simulink model "main_sim_adapt_Gref_SP"  (Simulink 7.2)
settings: Solver=ode2  SolverMode=SingleTasking  StartTime=0.0  StopTime=tsim_max  FixedStep=dtsim  RelTol=1e-3
StopFcn:
  | %mkplt
values from neighbouring files (symbols this model uses):
  aero_surf_qbar_off = get_value('aero_surf_qbar_off')    [setup_claw.m]
  aero_surf_qbar_on = get_value('aero_surf_qbar_on')    [setup_claw.m]
  assertion_time = get_value('assertion_time')    [setup_sim.m]
  att_cmd_select = get_value('att_cmd_select')    [setup_sim.m]
  att_trim_IC = orientation.att'    [setup_claw.m]
  att_type_numbers = cell2mat(struct2cell(att_type))    [setup_constants.m]
  chi_trim_IC = orientation.Vchigam(2)    [setup_claw.m]
  command_time = engage_time + 2.0    [setup_sim.m]
  compute_all_rate_cols = get_value('compute_all_rate_cols')    [setup_claw.m]
  compute_all_vel_cols = get_value('compute_all_vel_cols')    [setup_claw.m]
  da_trim_IC = tmp(1)    [setup_claw.m]
  dc_L2W_IC = orientation.dc_L2W    [setup_claw.m]
  de_trim_IC = tmp(2)    [setup_claw.m]
  dr_trim_IC = tmp(3)    [setup_claw.m]
  dtsim = get_value('dtsim')    [setup_sim.m]
  E_trim_IC = MACH_pos_IC(2)    [setup_claw.m]
  Ed_trim_IC = MACH_vel_IC(2)    [setup_claw.m]
  gain_set = gain_set_next    (= 1)    [setup_claw.m]
  gain_var_struct = rmfield(gain_var_struct,setdiff(fieldnames(gain_var_struct),{'name','size'}))    [setup_claw.m]
  gamma_trim_IC = orientation.Vchigam(3)    [setup_claw.m]
  h_trim_IC = MACH_pos_IC(3)    [setup_claw.m]
  hd_trim_IC = MACH_vel_IC(3)    [setup_claw.m]
  ideal_vel_Kb = MACH_vel_Kb(1)    [setup_sim.m]
  MACH = rmfield(MACH,'vel_throt_lrlim')    [setup_claw.m]
  MACH_att_fb = get_value('MACH_att_fb','onerror',0)    [setup_claw.m]
  MACH_att_int_IC = (1-MACH_att_Kc).*MACH_quat_IC'    [setup_ideal.m]
  MACH_att_Kb = repval(att_kbnom,MACH.att_num_cv)    [setup_claw.m]
  MACH_att_Kc = Ki2Kc(MACH_att_Ki)    [setup_ideal.m]
  MACH_att_Ki = repval(att_fi,MACH.att_num_cv)    [setup_claw.m]
  MACH_gain_mat = vertcat(MACH_gain_mat, this_gain_mat)    [setup_claw.m]
  MACH_mass_IC = obac_params.mass_IC    [setup_claw.m]
  MACH_pos_IC = x_obac_IC(MACH.NEh_idx)    [setup_claw.m]
  MACH_pos_int_IC = (1-MACH_pos_Kc).*MACH_pos_IC' + MACH_vel_IC'./MACH_pos_Kb    [setup_ideal.m]
  MACH_pos_Kb = repval(pos_kbnom,MACH.pos_num_cv)    [setup_claw.m]
  MACH_pos_Kc = Ki2Kc(MACH_pos_Ki)    [setup_ideal.m]
  MACH_pos_Ki = repval(pos_fi,MACH.pos_num_cv)    [setup_claw.m]
  MACH_pqr_Bmat_IC = Bo(MACH.pqr_idx,MACH.pqr_u_idx)    [setup_claw.m]
  MACH_pqr_IC = pqr_trim_IC    [setup_claw.m]
  MACH_pqr_int_IC = (1-MACH_pqr_Kc).*MACH_pqr_IC'    [setup_ideal.m]
  MACH_pqr_Kb = repval(pqr_kbnom,MACH.pqr_num_cv)    [setup_claw.m]
  MACH_pqr_Kc = Ki2Kc(MACH_pqr_Ki)    [setup_ideal.m]
  MACH_pqr_Ki = repval(pqr_fi,MACH.pqr_num_cv)    [setup_claw.m]
  MACH_pqr_u_IC = [ vanes_trim_IC; tvc_trim_IC; rcs_trim_IC ]    [setup_claw.m]
  MACH_quat_IC = quat_trim_IC    [setup_claw.m]
  MACH_throttle_IC = throttle_trim_IC    [setup_claw.m]
  MACH_U_nom_IC = zeros(MACH.num_u,1)    [setup_claw.m]
  MACH_vel_Bmat_IC = MACH_vel_Bmat_IC*inv(vel_perts)    [setup_claw.m]
  MACH_vel_cvdnom_IC = repval(get_value('vel_cvdnom_IC','onerror',MACH_vel_cvdnom_IC),length(MACH_vel_cvdnom_IC))'    [setup_claw.m]
  MACH_vel_IC = orientation.NdEdhd'    [setup_claw.m]
  MACH_vel_int_IC = (1-MACH_vel_Kc).*MACH_vel_IC'    [setup_ideal.m]
  MACH_vel_Kb = repval(vel_kbnom,MACH.vel_num_cv)    [setup_claw.m]
  MACH_vel_Kc = Ki2Kc(MACH_vel_Ki)    [setup_ideal.m]
  MACH_vel_Ki = repval(vel_fi,MACH.vel_num_cv)    [setup_claw.m]
  MACH_vel_uold_IC = [ MACH_quat_IC; MACH_throttle_IC ]    [setup_claw.m]
  N_trim_IC = MACH_pos_IC(1)    [setup_claw.m]
  Nd_trim_IC = MACH_vel_IC(1)    [setup_claw.m]
  obac_params = define_model('obac', get_value('obac_model_type'))    [setup_claw.m]
  pos_cmd_select = get_value('pos_cmd_select')    [setup_sim.m]
  pqr_trim_IC = [ 0 0 0 ]'    [setup_claw.m]
  rate_cmd_select = get_value('rate_cmd_select')    [setup_sim.m]
  rcs_cvddes_thresh = get_value('rcs_cvddes_thresh')    [setup_claw.m]
  reset_camcmd_on_entry = get_value('reset_camcmd_on_entry')    [setup_claw.m]
  throttle_trim_IC = u_obac_IC(MACH.throttle_idx)    [setup_claw.m]
  trac_params = define_model('trac', get_value('trac_model_type','onerror',obac_params.model_type))    [setup_sim.m]
  use_auto_att_type = get_value('use_auto_att_type','onerror',0)    [setup_claw.m]
  use_eow_as_iv = get_value('use_eow_as_iv')    [setup_claw.m]
  use_full_surf_cmd = get_value('use_full_surf_cmd')    [setup_sim.m]
  use_nav = get_value('use_nav')    [setup_claw.m]
  use_NdEdh_pos = get_value('use_NdEdh_pos')    [setup_claw.m]
  use_pos_fltpath_lim = get_value('use_pos_fltpath_lim')    [setup_claw.m]
  use_throt_estimate = get_value('use_throt_estimate')    [setup_claw.m]
  use_variable_mass = get_value('use_variable_mass')    [setup_claw.m]
  use_wind_est = get_value('use_wind_est')    [setup_claw.m]
  V_trim_IC = orientation.Vchigam(1)    [setup_claw.m]
  vel_cmd_ramp_time = get_value('vel_cmd_ramp_time')    [setup_claw.m]
  vel_cmd_select = get_value('vel_cmd_select')    [setup_sim.m]
  x_trac_IC = x_obac_IC    [setup_sim.m]
undefined symbols (not defined in the file or in its folder): accel_cmd, alpha_trim, Am, att_type, B1, bb_ellipsoid, bb_params, Bm, C, constants, cosA, DiscIntNeverNeededParam, DZkx, DZtheta, E_rwy, Ed_cmd, eow_boundary, flag_autoadapt, flag_exsig, flag_uad, full_surf_llim, full_surf_ulim, gam_cmd_descent, gam_cmd_preflare, gamdot_cmd_descent, gamdot_cmd_flare, gamdot_cmd_preflare, Gamtheta, Gamx, hd_cmd, in_error_thresh, in_exsig_vecin, in_exsig_vecout, in_reset_stoptime, in_t_exsig, in_t_timer, in_tadaptoff_forced, in_tadapton_forced, Kb, Kxhat0, Kxnom, Kxstar, max_chi_cmd, max_LOS_rate, max_vel_cmd, min_chi_cmd, min_vel_cmd, modes, N_rwy, Nd_cmd, Nrbf, P, pos, Sig, sinA, target_pos_IC, target_range_blind, target_range_detect, target_range_homing, target_vel_IC ... (+11)
libraries: simulink x44, utility_lib x36, mach_lib x24, model_lib x13, simulink_need_slupdate x8, models x8
(part 6 of 8)

== system main_sim_adapt_Gref_SP/claw_main/state est/process sensors/navigation complementary filter ==
  NEh nav : Inport  OutDataType=sfix(16)  OutScaling=2^0
  NEh dot : Inport  Port=2  OutDataType=sfix(16)  OutScaling=2^0
  Gain1 : Gain  Gain=MACH.K_velpos  ParameterDataType=sfix(16)  ParameterScaling=2^0  OutDataType=sfix(16)  OutScaling=2^0  SaturateOnIntegerOverflow=on  OutDataTypeStr=Inherit: Same as input  ParamDataTypeStr=Inherit: Same as input
  Sum1 : Sum  Inputs=|+-  OutDataType=sfix(16)  OutScaling=2^0  SaturateOnIntegerOverflow=on
  Sum2 : Sum  Inputs=++|  OutDataType=sfix(16)  OutScaling=2^0  SaturateOnIntegerOverflow=on  InputSameDT=on  OutDataTypeStr=Inherit: Same as first input
  integration1 : DiscreteIntegrator  SampleTime=-1  OutDataType=sfix(16)  OutScaling=2^0  ICPrevOutput=DiscIntNeverNeededParam  ICPrevScaledInput=DiscIntNeverNeededParam
  NEh_fil : Outport  OutDataType=sfix(16)  OutScaling=2^0
  wires:
  NEh dot/1 -> Sum2/1
  NEh nav/1 -> Sum1/1
  Gain1/1 -> Sum2/2
  Sum2/1 -> integration1/1
  integration1/1 -> NEh_fil/1, Sum1/2
  Sum1/1 -> Gain1/1

== system main_sim_adapt_Gref_SP/claw_main/state est/process sensors/select e sign ==
  e in : Inport  OutDataType=sfix(16)  OutScaling=2^0
  e_past : Inport  Port=2  OutDataType=sfix(16)  OutScaling=2^0
  Dot Product : simulink/Math Operations/Dot Product  InputSameDT=on  OutDataType=sfix(16)  OutScaling=2^-10  DoSatur=off
  Gain : Gain  Gain=-1  ParameterDataType=sfix(16)  ParameterScaling=2^0  OutDataType=sfix(16)  OutScaling=2^0  SaturateOnIntegerOverflow=on  OutDataTypeStr=Inherit: Same as input  ParamDataTypeStr=Inherit: Same as input
  Switch : Switch  SaturateOnIntegerOverflow=on
  e out : Outport  OutDataType=sfix(16)  OutScaling=2^0
  wires:
  e_past/1 -> Dot Product/2
  Switch/1 -> e out/1
  Gain/1 -> Switch/3
  Dot Product/1 -> Switch/2
  e in/1 -> Gain/1, Switch/1, Dot Product/1

== system main_sim_adapt_Gref_SP/claw_main/state est/process sensors/wait for valid nav ==
  latlonh : Inport  OutDataType=sfix(16)  OutScaling=2^0
  nav_ok : Inport  Port=2  OutDataType=sfix(16)  OutScaling=2^0
  Switch3 : Switch  Threshold=0.5  SaturateOnIntegerOverflow=on
  Unit Delay1 : UnitDelay  Orientation=left  SampleTime=-1
  LLh_0 : Outport  OutDataType=sfix(16)  OutScaling=2^0
  nav_valid : Outport  Port=2  OutDataType=sfix(16)  OutScaling=2^0
  wires:
  nav_ok/1 -> nav_valid/1, Switch3/2
  latlonh/1 -> Switch3/3
  Switch3/1 -> Unit Delay1/1, LLh_0/1
  Unit Delay1/1 -> Switch3/1

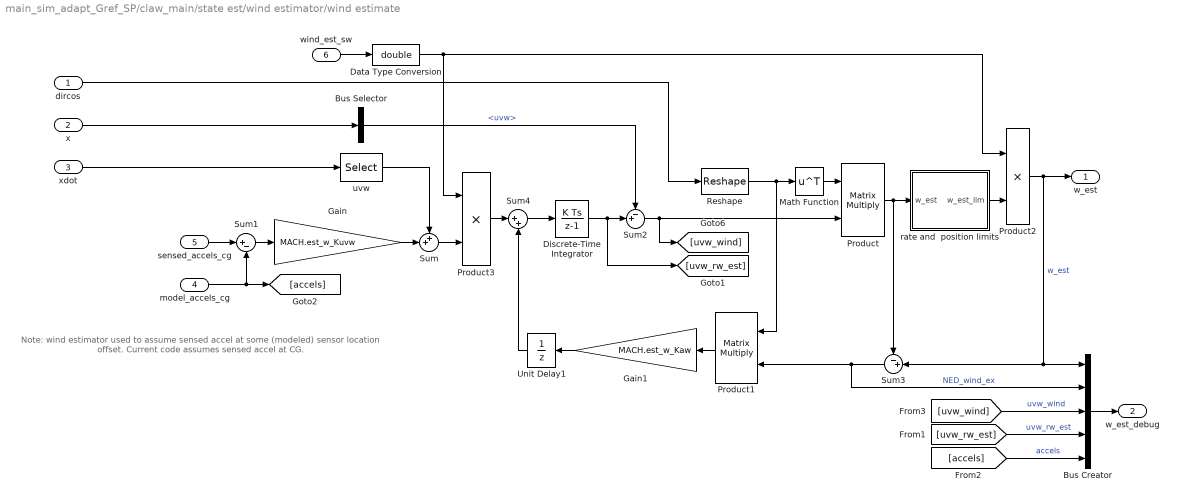
== system main_sim_adapt_Gref_SP/claw_main/state est/wind estimator/wind estimate ==
  note: Note: wind estimator used to assume sensed accel
      | at some (modeled) sensor location offset.
      |  Current code assumes sensed accel at CG.
  dircos : Inport  OutDataType=sfix(16)  OutScaling=2^0
  x : Inport  Port=2  OutDataType=sfix(16)  OutScaling=2^0
  xdot : Inport  Port=3  OutDataType=sfix(16)  OutScaling=2^0
  model_accels_cg : Inport  Port=4  OutDataType=sfix(16)  OutScaling=2^0
  sensed_accels_cg : Inport  Port=5  OutDataType=sfix(16)  OutScaling=2^0
  wind_est_sw : Inport  Port=6  OutDataType=sfix(16)  OutScaling=2^0
  Bus Creator : BusCreator  Inputs=5
  Bus Selector : BusSelector  OutputSignals=uvw
  Data Type Conversion : DataTypeConversion  OutDataTypeMode=double  OutDataType=sfix(16)  OutScaling=2^0  OutDataTypeStr=double  SaturateOnIntegerOverflow=on  RndMeth=Zero
  Discrete-Time Integrator : DiscreteIntegrator  SampleTime=-1  OutDataType=sfix(16)  OutScaling=2^0  ICPrevOutput=DiscIntNeverNeededParam  ICPrevScaledInput=DiscIntNeverNeededParam
  Gain : Gain  Gain=MACH.est_w_Kuvw  ParameterDataType=sfix(16)  ParameterScaling=2^0  OutDataType=sfix(16)  OutScaling=2^0  SaturateOnIntegerOverflow=on  OutDataTypeStr=Inherit: Same as input  ParamDataTypeStr=Inherit: Same as input
  Gain1 : Gain  Orientation=left  Gain=MACH.est_w_Kaw  ParameterDataType=sfix(16)  ParameterScaling=2^0  OutDataType=sfix(16)  OutScaling=2^0  SaturateOnIntegerOverflow=on  OutDataTypeStr=Inherit: Same as input  ParamDataTypeStr=Inherit: Same as input
  Math Function : Math  Operator=transpose  OutDataType=sfix(16)  OutScaling=2^0  SaturateOnIntegerOverflow=on
  Product : Product  Multiplication=Matrix(*)  OutDataType=sfix(16)  OutScaling=2^0  SaturateOnIntegerOverflow=on  OutDataTypeStr=Inherit: Same as first input
  Product1 : Product  Orientation=left  Multiplication=Matrix(*)  OutDataType=sfix(16)  OutScaling=2^0  SaturateOnIntegerOverflow=on  OutDataTypeStr=Inherit: Same as first input
  Product2 : Product  OutDataType=sfix(16)  OutScaling=2^0  SaturateOnIntegerOverflow=on  OutDataTypeStr=Inherit: Same as first input
  Product3 : Product  OutDataType=sfix(16)  OutScaling=2^0  SaturateOnIntegerOverflow=on  OutDataTypeStr=Inherit: Same as first input
  Reshape : Reshape  OutputDimensionality=Customize  OutputDimensions=[3,3]
  Sum : Sum  Inputs=++|  OutDataType=sfix(16)  OutScaling=2^0  SaturateOnIntegerOverflow=on  InputSameDT=on  OutDataTypeStr=Inherit: Same as first input
  Sum1 : Sum  Inputs=|+-  OutDataType=sfix(16)  OutScaling=2^0  SaturateOnIntegerOverflow=on  InputSameDT=on  OutDataTypeStr=Inherit: Same as first input
  Sum2 : Sum  Inputs=-+|  OutDataType=sfix(16)  OutScaling=2^0  SaturateOnIntegerOverflow=on
  Sum3 : Sum  Orientation=left  Inputs=-+|  OutDataType=sfix(16)  OutScaling=2^0  SaturateOnIntegerOverflow=on
  Sum4 : Sum  Inputs=|++  OutDataType=sfix(16)  OutScaling=2^0  SaturateOnIntegerOverflow=on  InputSameDT=on  OutDataTypeStr=Inherit: Same as first input
  Unit Delay1 : UnitDelay  Orientation=left  X0=zeros(3,1)  SampleTime=-1
  rate and  position limits : Subsystem
  uvw : Selector  InputPortWidth=MACH.num_x  IndexOptions=Index vector (dialog)  Indices=MACH.uvw_idx  OutputSizes=1
  w_est : Outport  OutDataType=sfix(16)  OutScaling=2^0
  w_est_debug : Outport  Port=2  OutDataType=sfix(16)  OutScaling=2^0
  wires:
  Discrete-Time Integrator/1 -> Sum2/2, [uvw_rw_est]
  sensed_accels_cg/1 -> Sum1/1
  Sum1/1 -> Gain/1
  Sum/1 -> Product3/2
  Gain/1 -> Sum/2
  Bus Selector/1 -> Sum2/1  "<uvw>"
  dircos/1 -> Reshape/1
  Reshape/1 -> Math Function/1, Product1/1
  Product/1 -> Sum3/1, rate and  position limits/1(w_est)
  Math Function/1 -> Product/1
  Sum2/1 -> Product/2, [uvw_wind]
  Gain1/1 -> Unit Delay1/1
  xdot/1 -> uvw/1
  uvw/1 -> Sum/1
  x/1 -> Bus Selector/1
  rate and  position limits/1(w_est_lim) -> Product2/2
  Product1/1 -> Gain1/1
  Sum3/1 -> Product1/2, Bus Creator/2  "NED_wind_ex"
  Product2/1 -> w_est/1, Sum3/2, Bus Creator/1  "w_est"
  wind_est_sw/1 -> Data Type Conversion/1
  Sum4/1 -> Discrete-Time Integrator/1
  Product3/1 -> Sum4/1
  Unit Delay1/1 -> Sum4/2
  Data Type Conversion/1 -> Product2/1, Product3/1
  [uvw_wind] -> Bus Creator/3  "uvw_wind"
  [uvw_rw_est] -> Bus Creator/4  "uvw_rw_est"
  [accels] -> Bus Creator/5  "accels"
  Bus Creator/1 -> w_est_debug/1
  model_accels_cg/1 -> Sum1/2, [accels]

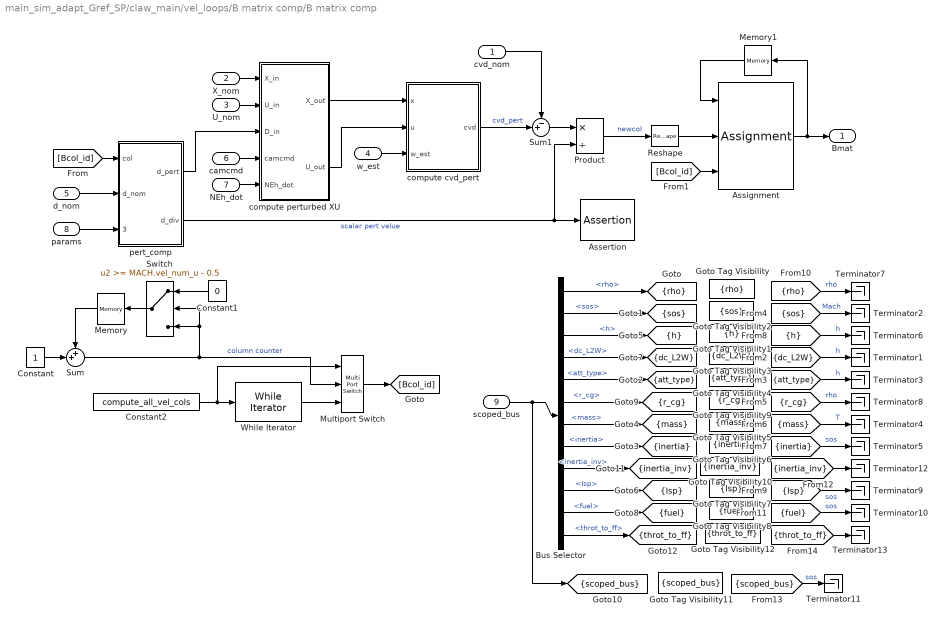
== system main_sim_adapt_Gref_SP/claw_main/vel_loops/B matrix comp/B matrix comp ==
  cvd_nom : Inport  OutDataType=sfix(16)  OutScaling=2^0
  X_nom : Inport  Port=2  OutDataType=sfix(16)  OutScaling=2^0
  U_nom : Inport  Port=3  OutDataType=sfix(16)  OutScaling=2^0
  w_est : Inport  Port=4  OutDataType=sfix(16)  OutScaling=2^0
  d_nom : Inport  Port=5  OutDataType=sfix(16)  OutScaling=2^0
  camcmd : Inport  Port=6  OutDataType=sfix(16)  OutScaling=2^0
  NEh_dot : Inport  Port=7  OutDataType=sfix(16)  OutScaling=2^0
  params : Inport  Port=8  OutDataType=sfix(16)  OutScaling=2^0
  scoped_bus : Inport  Port=9  OutDataType=sfix(16)  OutScaling=2^0
  Assertion : Assertion  Enabled=on
  Assignment : Assignment  NumberOfDimensions=2  IndexOptions=Assign all,Index vector (port)  Indices=-1,1  OutputSizes=1,1
  Bus Selector : BusSelector  OutputSignals=atmos_env.rho,atmos_env.sos,atmos_env.h,dc_L2W,att_type,mass_props.r_cg,mass_props.mass,mass_props.inertia,mass_props.inertia_inv,mass_props.Isp,mass_props.fuel,mass_props.throt_to_ff
  Constant : Constant  OutDataType=sfix(16)  OutScaling=2^0
  Constant1 : Constant  Orientation=left  Value=0  OutDataType=sfix(16)  OutScaling=2^0
  Constant2 : Constant  Value=compute_all_vel_cols  OutDataType=sfix(16)  OutScaling=2^0
  Goto Tag Visibility : GotoTagVisibility  GotoTag=rho
  Goto Tag Visibility1 : GotoTagVisibility  GotoTag=h
  Goto Tag Visibility10 : GotoTagVisibility  GotoTag=inertia_inv
  Goto Tag Visibility11 : GotoTagVisibility  GotoTag=scoped_bus
  Goto Tag Visibility12 : GotoTagVisibility  GotoTag=throt_to_ff
  Goto Tag Visibility2 : GotoTagVisibility  GotoTag=sos
  Goto Tag Visibility3 : GotoTagVisibility  GotoTag=dc_L2W
  Goto Tag Visibility4 : GotoTagVisibility  GotoTag=att_type
  Goto Tag Visibility5 : GotoTagVisibility  GotoTag=mass
  Goto Tag Visibility6 : GotoTagVisibility  GotoTag=inertia
  Goto Tag Visibility7 : GotoTagVisibility  GotoTag=Isp
  Goto Tag Visibility8 : GotoTagVisibility  GotoTag=fuel
  Goto Tag Visibility9 : GotoTagVisibility  GotoTag=r_cg
  Memory : Memory  Orientation=left  InheritSampleTime=on
  Memory1 : Memory  Orientation=left  X0=MACH_vel_Bmat_IC  InheritSampleTime=on
  Multiport Switch : MultiPortSwitch  Inputs=2  zeroidx=on
  Product : Product  Inputs=*/  OutDataType=sfix(16)  OutScaling=2^0  SaturateOnIntegerOverflow=on  InputSameDT=on  OutDataTypeStr=Inherit: Same as first input
  Reshape : Reshape  OutputDimensionality=Column vector (2-D)
  Sum : Sum  Inputs=++|  OutDataType=sfix(16)  OutScaling=2^0  SaturateOnIntegerOverflow=on  InputSameDT=on  OutDataTypeStr=Inherit: Same as first input
  Sum1 : Sum  Inputs=-+|  OutDataType=sfix(16)  OutScaling=2^0  SaturateOnIntegerOverflow=on  InputSameDT=on  OutDataTypeStr=Inherit: Same as first input
  Switch : Switch  Orientation=left  Threshold=MACH.vel_num_u - 0.5  SaturateOnIntegerOverflow=on  InputSameDT=on
  Terminator{1..13} (13 alike) : Terminator
  While Iterator : WhileIterator  MaxIters=MACH.vel_num_u  WhileBlockType=do-while  ShowIterationPort=on
  compute cvd_pert : Subsystem
  compute perturbed XU : Subsystem
  pert_comp : Subsystem
  Bmat : Outport  OutDataType=sfix(16)  OutScaling=2^0
  tag scope: Isp=scoped, att_type=scoped, dc_L2W=scoped, fuel=scoped, h=scoped, inertia=scoped, inertia_inv=scoped, mass=scoped, r_cg=scoped, rho=scoped, scoped_bus=scoped, sos=scoped, throt_to_ff=scoped
  wires:
  U_nom/1 -> compute perturbed XU/2(U_in)
  X_nom/1 -> compute perturbed XU/1(X_in)
  Product/1 -> Reshape/1  "newcol"
  Sum1/1 -> Product/1
  [Bcol_id] -> Assignment/3
  Reshape/1 -> Assignment/2
  Assignment/1 -> Bmat/1, Memory1/1
  [Bcol_id] -> pert_comp/1(col)
  d_nom/1 -> pert_comp/2(d_nom)
  pert_comp/2(d_div) -> Product/2, Assertion/1  "scalar pert value"
  pert_comp/1(d_pert) -> compute perturbed XU/3(D_in)
  w_est/1 -> compute cvd_pert/3(w_est)
  camcmd/1 -> compute perturbed XU/4(camcmd)
  NEh_dot/1 -> compute perturbed XU/5(NEh_dot)
  compute perturbed XU/1(X_out) -> compute cvd_pert/1(x)
  params/1 -> pert_comp/3(params)
  compute perturbed XU/2(U_out) -> compute cvd_pert/2(u)
  Memory1/1 -> Assignment/1
  scoped_bus/1 -> Bus Selector/1, [scoped_bus]
  [rho] -> Terminator7/1  "rho"
  [sos] -> Terminator2/1  "Mach"
  [h] -> Terminator6/1  "h"
  Bus Selector/1 -> [rho]  "<rho>"
  Bus Selector/2 -> [sos]  "<sos>"
  Bus Selector/3 -> [h]  "<h>"
  [dc_L2W] -> Terminator1/1  "h"
  Bus Selector/4 -> [dc_L2W]  "<dc_L2W>"
  Constant2/1 -> Multiport Switch/1, While Iterator/1
  While Iterator/1 -> Multiport Switch/3
  Constant1/1 -> Switch/1
  Sum/1 -> Switch/3, Switch/2, Multiport Switch/2  "column counter"
  Switch/1 -> Memory/1
  Memory/1 -> Sum/1
  Constant/1 -> Sum/2
  Multiport Switch/1 -> [Bcol_id]
  [att_type] -> Terminator3/1  "h"
  Bus Selector/5 -> [att_type]  "<att_type>"
  [r_cg] -> Terminator8/1  "rho"
  [mass] -> Terminator4/1  "T"
  [inertia] -> Terminator5/1  "sos"
  Bus Selector/6 -> [r_cg]  "<r_cg>"
  Bus Selector/7 -> [mass]  "<mass>"
  Bus Selector/8 -> [inertia]  "<inertia>"
  [Isp] -> Terminator9/1  "sos"
  Bus Selector/10 -> [Isp]  "<Isp>"
  [fuel] -> Terminator10/1  "sos"
  Bus Selector/11 -> [fuel]  "<fuel>"
  compute cvd_pert/1(cvd) -> Sum1/2  "cvd_pert"
  cvd_nom/1 -> Sum1/1
  [inertia_inv] -> Terminator12/1
  Bus Selector/9 -> [inertia_inv]  "<inertia_inv>"
  [scoped_bus] -> Terminator11/1  "sos"
  Bus Selector/12 -> [throt_to_ff]  "<throt_to_ff>"
  [throt_to_ff] -> Terminator13/1

== system main_sim_adapt_Gref_SP/claw_main/vel_loops/B matrix comp/compute cvd_nom ==
  note: Note: this computation of NEh accelerations
      | assumes that pqr = 0
  x : Inport  OutDataType=sfix(16)  OutScaling=2^0
  u : Inport  Port=2  OutDataType=sfix(16)  OutScaling=2^0
  w_est : Inport  Port=3  OutDataType=sfix(16)  OutScaling=2^0
  Bus Selector : BusSelector  OutputSignals=dircos
  Gain : Gain  Gain=[1 1 -1]  ParameterDataType=sfix(16)  ParameterScaling=2^0  OutDataType=sfix(16)  OutScaling=2^0  SaturateOnIntegerOverflow=on  OutDataTypeStr=Inherit: Same as input  ParamDataTypeStr=Inherit: Same as input
  Math Function : Math  Operator=transpose  OutDataType=sfix(16)  OutScaling=2^0  SaturateOnIntegerOverflow=on
  Product : Product  Multiplication=Matrix(*)  OutDataType=sfix(16)  OutScaling=2^0  SaturateOnIntegerOverflow=on  InputSameDT=on  OutDataTypeStr=Inherit: Same as first input
  Reshape : Reshape  OutputDimensionality=Customize  OutputDimensions=[3,3]
  cl model : models/gtm-obac  SystemSampleTime=-1
  uvw_dot : Selector  InputPortWidth=MACH.num_x  IndexOptions=Index vector (dialog)  Indices=MACH.uvw_idx  OutputSizes=1
  cvd : Outport  OutDataType=sfix(16)  OutScaling=2^0
  wires:
  uvw_dot/1 -> Product/2
  x/1 -> cl model/1
  Reshape/1 -> Math Function/1
  Math Function/1 -> Product/1
  Product/1 -> Gain/1
  Gain/1 -> cvd/1
  Bus Selector/1 -> Reshape/1  "<dircos>"
  u/1 -> cl model/2
  w_est/1 -> cl model/3
  cl model/1 -> uvw_dot/1
  cl model/2 -> Bus Selector/1

== system main_sim_adapt_Gref_SP/claw_main/vel_loops/B matrix comp/compute nominal XU ==
  X_in : Inport  OutDataType=sfix(16)  OutScaling=2^0
  U_in : Inport  Port=2  OutDataType=sfix(16)  OutScaling=2^0
  D_in : Inport  Port=3  OutDataType=sfix(16)  OutScaling=2^0
  camcmd : Inport  Port=4  OutDataType=sfix(16)  OutScaling=2^0
  NEh_dot : Inport  Port=5  OutDataType=sfix(16)  OutScaling=2^0
  Assignment1 : Assignment  IndexOptions=Index vector (dialog)  Indices=MACH.throttle_idx  OutputSizes=[1 1]
  Assignment2 : Assignment  IndexOptions=Index vector (dialog)  Indices=[ MACH.quat_idx MACH.uvw_idx]  OutputSizes=[1 1]
  Demux1 : Demux  Outputs=[ 2 MACH.num_u_throt ]
  Gain : Gain  Gain=[1 1 -1]  ParameterDataType=sfix(16)  ParameterScaling=2^0  OutDataType=sfix(16)  OutScaling=2^0  SaturateOnIntegerOverflow=on  OutDataTypeStr=Inherit: Same as input  ParamDataTypeStr=Inherit: Same as input
  Mux : Mux  Inputs=[ 2 1 ]
  Mux1 : Mux  Inputs=2
  Product1 : Product  Multiplication=Matrix(*)  OutDataType=sfix(16)  OutScaling=2^0  SaturateOnIntegerOverflow=on  OutDataTypeStr=Inherit: Same as first input
  Reshape1 : Reshape  OutputDimensionality=Customize  OutputDimensions=[3,3]
  Selector1 : Selector  InputPortWidth=MACH.num_x  IndexOptions=Index vector (dialog)  Indices=MACH.quat_idx  OutputSizes=1
  att2dc : utility_lib/att2dc  SystemSampleTime=-1
  dc2e_ref : utility_lib/dc2e_ref  SystemSampleTime=-1
  X_out : Outport  OutDataType=sfix(16)  OutScaling=2^0
  U_out : Outport  Port=2  OutDataType=sfix(16)  OutScaling=2^0
  wires:
  Mux/1 -> att2dc/1
  Demux1/2 -> Assignment1/2  "throttle"
  D_in/1 -> Demux1/1
  U_in/1 -> Assignment1/1
  X_in/1 -> Assignment2/1, Selector1/1
  Assignment1/1 -> U_out/1
  camcmd/1 -> Mux/2
  Demux1/1 -> Mux/1
  NEh_dot/1 -> Gain/1
  Reshape1/1 -> Product1/1
  Assignment2/1 -> X_out/1
  att2dc/1 -> Reshape1/1, dc2e_ref/1
  dc2e_ref/1 -> Mux1/1  "e"
  Gain/1 -> Product1/2  "NED_dot"
  Selector1/1 -> dc2e_ref/2
  Product1/1 -> Mux1/2  "uvw"
  Mux1/1 -> Assignment2/2

== system main_sim_adapt_Gref_SP/claw_main/vel_loops/convert accel_cmd to NED_dd_cmd/NED_dd cmd ==
  NEH_dd_cmd_in : Inport  OutDataType=sfix(16)  OutScaling=2^0
  Action Port : ActionPort  ActionType=case
  NEh_dd_cmd : Outport  OutDataType=sfix(16)  OutScaling=2^0  InitialOutput=zeros(3,1)
  wires:
  NEH_dd_cmd_in/1 -> NEh_dd_cmd/1

== system main_sim_adapt_Gref_SP/claw_main/vel_loops/convert accel_cmd to NED_dd_cmd/vchigam_dot cmd ==
  vchigam_dot_cmd : Inport  OutDataType=sfix(16)  OutScaling=2^0
  NEh_d : Inport  Port=2  OutDataType=sfix(16)  OutScaling=2^0
  Action Port : ActionPort  ActionType=case
  Math Function : Math  Operator=transpose  OutDataType=sfix(16)  OutScaling=2^0  SaturateOnIntegerOverflow=on
  Product2 : Product  Multiplication=Matrix(*)  OutDataType=sfix(16)  OutScaling=2^0  RndMeth=Zero
  Reshape1 : Reshape  OutputDimensionality=Customize  OutputDimensions=[3 3]
  convert to NED_d : Gain  Gain=[1 1 -1]  ParameterDataType=sfix(16)  ParameterScaling=2^0  OutDataType=sfix(16)  OutScaling=2^0
  convert to NEh_dd : Gain  Gain=[1 1 -1]  ParameterDataType=sfix(16)  ParameterScaling=2^0  OutDataType=sfix(16)  OutScaling=2^0
  polar to cart : Subsystem
  vec2dc : utility_lib/vec2dc  SystemSampleTime=-1
  NEh_dd_cmd : Outport  OutDataType=sfix(16)  OutScaling=2^0  InitialOutput=zeros(3,1)
  wires:
  vec2dc/1 -> Reshape1/1
  Reshape1/1 -> Math Function/1
  convert to NED_d/1 -> vec2dc/1
  polar to cart/1(along_dd;cross_dd;vert_dd) -> Product2/2
  NEh_d/1 -> convert to NED_d/1
  Product2/1 -> convert to NEh_dd/1
  convert to NEh_dd/1 -> NEh_dd_cmd/1
  Math Function/1 -> Product2/1
  vchigam_dot_cmd/1 -> polar to cart/2(vchigam_dot_cmd)
  vec2dc/2 -> polar to cart/1(scaling_info)

== system main_sim_adapt_Gref_SP/claw_main/vel_loops/set di params/att limits ==
  uvw : Inport  OutDataType=sfix(16)  OutScaling=2^0
  Bus Creator : BusCreator
  Constant : Constant  Value=MACH.vel_att_ulim  VectorParams1D=off  OutDataType=sfix(16)  OutScaling=2^0
  Constant1 : Constant  Value=MACH.vel_att_lrlim  OutDataType=sfix(16)  OutScaling=2^0
  Constant2 : Constant  Value=MACH.vel_att_urlim  OutDataType=sfix(16)  OutScaling=2^0
  Constant3 : Constant  Value=MACH.az_ulim  OutDataType=sfix(16)  OutScaling=2^0
  Constant7 : Constant  Value=MACH.vel_att_llim  VectorParams1D=off  OutDataType=sfix(16)  OutScaling=2^0
  Constant8 : Constant  Value=MACH.az_llim  OutDataType=sfix(16)  OutScaling=2^0
  Reshape1 : Reshape
  Reshape3 : Reshape
  Selector1 : Selector  NumberOfDimensions=2  InputPortWidth=3  IndexOptions=Index vector (port),Select all  Indices=1,-1  OutputSizes=1
  Selector2 : Selector  NumberOfDimensions=2  InputPortWidth=3  IndexOptions=Index vector (port),Select all  Indices=1,-1  OutputSizes=1
  velocity based angular rate llim : mach_lib/velocity based angular rate limit  SystemSampleTime=-1  q_idx=2
  velocity based angular rate ulim : mach_lib/velocity based angular rate limit  SystemSampleTime=-1  q_idx=2
  att_limits : Outport  OutDataType=sfix(16)  OutScaling=2^0
  wires:
  [att_type] -> Selector1/2, Selector2/2
  Constant/1 -> Selector1/1
  Constant7/1 -> Selector2/1
  Selector1/1 -> Reshape1/1
  Selector2/1 -> Reshape3/1
  Reshape1/1 -> Bus Creator/1  "att_ulim"
  Reshape3/1 -> Bus Creator/2  "att_llim"
  Constant2/1 -> velocity based angular rate ulim/1
  Constant8/1 -> velocity based angular rate ulim/2
  Constant1/1 -> velocity based angular rate llim/1
  Constant3/1 -> velocity based angular rate llim/2
  uvw/1 -> velocity based angular rate ulim/3, velocity based angular rate llim/3
  velocity based angular rate ulim/1 -> Bus Creator/3  "att_urlim"
  velocity based angular rate llim/1 -> Bus Creator/4  "att_lrlim"
  Bus Creator/1 -> att_limits/1

== system main_sim_adapt_Gref_SP/claw_main/vel_loops/set di params/combine limits ==
  att_limits : Inport  OutDataType=sfix(16)  OutScaling=2^0
  throt_limits : Inport  Port=2  OutDataType=sfix(16)  OutScaling=2^0
  Bus Creator : BusCreator
  Bus Selector : BusSelector  OutputSignals=att_ulim,att_llim,att_urlim,att_lrlim
  Bus Selector1 : BusSelector  OutputSignals=throt_ulim,throt_llim,throt_urlim,throt_lrlim
  Mux{,1..3} (4 alike) : Mux  Inputs=2
  vel_u_limits : Outport  OutDataType=sfix(16)  OutScaling=2^0
  wires:
  att_limits/1 -> Bus Selector/1
  throt_limits/1 -> Bus Selector1/1
  Bus Selector/1 -> Mux/1  "<att_ulim>"
  Bus Selector/2 -> Mux1/1  "<att_llim>"
  Bus Selector/3 -> Mux2/1  "<att_urlim>"
  Bus Selector/4 -> Mux3/1  "<att_lrlim>"
  Bus Selector1/1 -> Mux/2  "<throt_ulim>"
  Bus Selector1/2 -> Mux1/2  "<throt_llim>"
  Bus Selector1/3 -> Mux2/2  "<throt_urlim>"
  Bus Selector1/4 -> Mux3/2  "<throt_lrlim>"
  Mux/1 -> Bus Creator/1  "u_ulim"
  Mux1/1 -> Bus Creator/2  "u_llim"
  Mux2/1 -> Bus Creator/3  "u_urlim"
  Mux3/1 -> Bus Creator/4  "u_lrlim"
  Bus Creator/1 -> vel_u_limits/1

== system main_sim_adapt_Gref_SP/claw_main/vel_loops/set di params/compute dc_fltpath ==
  NEh_dot_fltpath : Inport  OutDataType=sfix(16)  OutScaling=2^0
  Gain : Gain  Gain=repmat([1 1 -1],3,1)  ParameterDataType=sfix(16)  ParameterScaling=2^0  OutDataType=sfix(16)  OutScaling=2^0
  Gain1 : Gain  Gain=[1 1 -1]  ParameterDataType=sfix(16)  ParameterScaling=2^0  OutDataType=sfix(16)  OutScaling=2^0
  Reshape : Reshape  OutputDimensionality=Customize  OutputDimensions=[3 3]
  Terminator : Terminator
  vec2dc : utility_lib/vec2dc  SystemSampleTime=-1
  dc_fltpath : Outport  OutDataType=sfix(16)  OutScaling=2^0
  wires:
  vec2dc/1 -> Reshape/1
  Reshape/1 -> Gain/1
  Gain1/1 -> vec2dc/1
  vec2dc/2 -> Terminator/1
  Gain/1 -> dc_fltpath/1
  NEh_dot_fltpath/1 -> Gain1/1

== system main_sim_adapt_Gref_SP/claw_main/vel_loops/set di params/throttle limits ==
  full_surf : Inport  OutDataType=sfix(16)  OutScaling=2^0
  throt_old : Inport  Port=2  OutDataType=sfix(16)  OutScaling=2^0
  Bus Creator : BusCreator
  Bus Selector1 : BusSelector  OutputSignals=full_surf_ulim,full_surf_llim,full_surf_urlim,full_surf_lrlim
  Selector{1..2,5..6} (4 alike) : Selector  InputPortWidth=MACH.num_u  IndexOptions=Index vector (dialog)  Indices=MACH.throttle_idx  OutputSizes=1
  rate limit limits : mach_lib/rate limit limits  SystemSampleTime=-1  ulim=MACH.vel_throt_ulim  llim=MACH.vel_throt_llim
  throt_limits : Outport  OutDataType=sfix(16)  OutScaling=2^0
  wires:
  Bus Selector1/1 -> Selector5/1  "<full_surf_ulim>"
  Bus Selector1/2 -> Selector6/1  "<full_surf_llim>"
  full_surf/1 -> Bus Selector1/1
  throt_old/1 -> rate limit limits/1
  Selector5/1 -> rate limit limits/2
  Selector6/1 -> rate limit limits/3
  Bus Creator/1 -> throt_limits/1
  rate limit limits/1 -> Bus Creator/1  "throt_ulim"
  rate limit limits/2 -> Bus Creator/2  "throt_llim"
  Bus Selector1/3 -> Selector1/1  "<full_surf_urlim>"
  Bus Selector1/4 -> Selector2/1  "<full_surf_lrlim>"
  Selector1/1 -> rate limit limits/4, Bus Creator/3  "throt_urlim"
  Selector2/1 -> rate limit limits/5, Bus Creator/4  "throt_lrlim"

== system main_sim_adapt_Gref_SP/control input (modified)/control input/form control input/add effector control params ==
  full_surf_cmd : Inport  OutDataType=sfix(16)  OutScaling=2^0
  Bus Creator : BusCreator  Inputs=9
  From Workspace : FromWorkspace  VariableName=full_surf_limits_fw.obac.ulim  SampleTime=MACH.dt  Interpolate=off  OutputAfterFinalValue=Holding final value
  From Workspace1 : FromWorkspace  VariableName=full_surf_limits_fw.obac.llim  SampleTime=MACH.dt  Interpolate=off  OutputAfterFinalValue=Holding final value
  From Workspace2 : FromWorkspace  VariableName=full_surf_limits_fw.obac.limit_select  SampleTime=MACH.dt  Interpolate=off  OutputAfterFinalValue=Holding final value
  From Workspace3 : FromWorkspace  VariableName=full_surf_limits_fw.obac.urlim  SampleTime=MACH.dt  Interpolate=off  OutputAfterFinalValue=Holding final value
  From Workspace4 : FromWorkspace  VariableName=full_surf_limits_fw.obac.lrlim  SampleTime=MACH.dt  Interpolate=off  OutputAfterFinalValue=Holding final value
  From Workspace5 : FromWorkspace  VariableName=full_surf_limits_fw.obac.pref_select  SampleTime=MACH.dt  Interpolate=off  OutputAfterFinalValue=Holding final value
  From Workspace6 : FromWorkspace  VariableName=full_surf_limits_fw.obac.pref  SampleTime=MACH.dt  Interpolate=off  OutputAfterFinalValue=Holding final value
  From Workspace7 : FromWorkspace  VariableName=full_surf_limits_fw.obac.pref_wght  SampleTime=MACH.dt  Interpolate=off  OutputAfterFinalValue=Holding final value
  full_surf : Outport  OutDataType=sfix(16)  OutScaling=2^0
  wires:
  From Workspace1/1 -> Bus Creator/3  "full_surf_llim"
  From Workspace/1 -> Bus Creator/2  "full_surf_ulim"
  full_surf_cmd/1 -> Bus Creator/1  "full_surf_cmd"
  Bus Creator/1 -> full_surf/1
  From Workspace3/1 -> Bus Creator/4  "full_surf_urlim"
  From Workspace4/1 -> Bus Creator/5  "full_surf_lrlim"
  From Workspace2/1 -> Bus Creator/6  "full_surf_lock"
  From Workspace5/1 -> Bus Creator/7  "full_surf_pref_select"
  From Workspace6/1 -> Bus Creator/8  "full_surf_pref"
  From Workspace7/1 -> Bus Creator/9  "full_surf_pref_wght"

== system main_sim_adapt_Gref_SP/control input (modified)/control input/form control input/engine parameters ==
  Bus Creator2 : BusCreator  Inputs=3
  Constant : Constant  Value=obac_params.Isp_sl  OutDataType=sfix(16)  OutScaling=2^0
  Constant1 : Constant  Value=obac_params.Isp_vacuum  OutDataType=sfix(16)  OutScaling=2^0
  Constant2 : Constant  Value=obac_params.throt_to_ff  OutDataType=sfix(16)  OutScaling=2^0
  engines : Outport  OutDataType=sfix(16)  OutScaling=2^0
  wires:
  Constant1/1 -> Bus Creator2/2  "Isp_vacuum"
  Constant/1 -> Bus Creator2/1  "Isp_sl"
  Bus Creator2/1 -> engines/1
  Constant2/1 -> Bus Creator2/3  "throt_to_ff"

== system main_sim_adapt_Gref_SP/control input (modified)/control input/form control input/mode switches ==
  control_input : Inport  OutDataType=sfix(16)  OutScaling=2^0
  Bus Creator1 : BusCreator  Inputs=17
  Bus Selector4 : BusSelector  OutputSignals=CLAW_mode,accel_submode
  Compare To Zero : simulink/Logic and Bit Operations/Compare To Zero  SystemSampleTime=-1  relop=>  LogicOutDataTypeMode=boolean  ZeroCross=off
  Data Type Conversion : DataTypeConversion  OutDataType=sfix(16)  OutScaling=2^0
  From Workspace : FromWorkspace  VariableName=enable_bb_fw  SampleTime=MACH.dt  Interpolate=off  OutputAfterFinalValue=Holding final value
  From Workspace1 : FromWorkspace  VariableName=use_att_rate_cmd_fw  SampleTime=MACH.dt  Interpolate=off  OutputAfterFinalValue=Holding final value
  From Workspace2 : FromWorkspace  VariableName=use_cam_rate_cmd_fw  SampleTime=MACH.dt  Interpolate=off  OutputAfterFinalValue=Holding final value
  From Workspace3 : FromWorkspace  VariableName=enable_homing_fw  SampleTime=MACH.dt  Interpolate=off  OutputAfterFinalValue=Holding final value
  From Workspace4 : FromWorkspace  VariableName=nav_enable_fw  SampleTime=MACH.dt  Interpolate=off  OutputAfterFinalValue=Holding final value
  From Workspace5 : FromWorkspace  VariableName=gain_set_fw  SampleTime=MACH.dt  Interpolate=off  OutputAfterFinalValue=Holding final value
  From Workspace6 : FromWorkspace  VariableName=att_type_fw  SampleTime=MACH.dt  Interpolate=off  OutputAfterFinalValue=Holding final value
  From Workspace7 : FromWorkspace  VariableName=use_held_aero_obac_fw  SampleTime=MACH.dt  Interpolate=off  OutputAfterFinalValue=Holding final value
  int_reset_sw : Constant  Value=0  OutDataType=sfix(16)  OutScaling=2^0
  llh_input_sw : Constant  Value=0  OutDataType=sfix(16)  OutScaling=2^0
  pre_takeoff_sw : Constant  Value=0  OutDataType=sfix(16)  OutScaling=2^0
  reset_pos_sw : Constant  Value=0  OutDataType=sfix(16)  OutScaling=2^0
  use_full_surf_cmd_sw : Constant  Value=use_full_surf_cmd  OutDataType=sfix(16)  OutScaling=2^0
  wind_est_sw : Constant  Value=0  OutDataType=sfix(16)  OutScaling=2^0
  mode_sw : Outport  OutDataType=sfix(16)  OutScaling=2^0
  wires:
  reset_pos_sw/1 -> Bus Creator1/5  "reset_pos_sw"
  wind_est_sw/1 -> Bus Creator1/6  "wind_est_sw"
  llh_input_sw/1 -> Bus Creator1/7  "llh_input_sw"
  Compare To Zero/1 -> Data Type Conversion/1  "engaged_sw"
  pre_takeoff_sw/1 -> Bus Creator1/4  "pre_takeoff_sw"
  int_reset_sw/1 -> Bus Creator1/8  "int_reset_sw"
  Data Type Conversion/1 -> Bus Creator1/2  "engaged_sw"
  use_full_surf_cmd_sw/1 -> Bus Creator1/11  "full_surf_cmd_sw"
  From Workspace2/1 -> Bus Creator1/10  "cam_rate_cmd_sw"
  From Workspace6/1 -> Bus Creator1/9  "att_type"
  From Workspace3/1 -> Bus Creator1/12  "enable_homing_sw"
  From Workspace1/1 -> Bus Creator1/13  "att_rate_cmd_sw"
  From Workspace4/1 -> Bus Creator1/14  "nav_enable_sw"
  From Workspace/1 -> Bus Creator1/15  "enable_bb_sw"
  From Workspace5/1 -> Bus Creator1/16  "gain_set_sw"
  From Workspace7/1 -> Bus Creator1/17  "use_held_aero_obac_sw"
  Bus Selector4/2 -> Bus Creator1/3  "<accel_submode>"
  Bus Creator1/1 -> mode_sw/1
  control_input/1 -> Bus Selector4/1
  Bus Selector4/1 -> Compare To Zero/1, Bus Creator1/1  "<CLAW_mode>"

== system main_sim_adapt_Gref_SP/control input (modified)/control input/form control input/select command ==
  cmd_bus : Inport  OutDataType=sfix(16)  OutScaling=2^0
  Bus Creator1 : BusCreator
  Bus Selector : BusSelector  OutputSignals=da_cmd,de_cmd,dr_cmd,throttle_cmd  OutputAsBus=on
  Bus Selector4 : BusSelector  OutputSignals=full_surf_cmd,accel_submode,CLAW_mode
  Multiport Switch : MultiPortSwitch  Inputs=5  zeroidx=on  SaturateOnIntegerOverflow=on
  att cmd select : Subsystem
  pos cmd select : Subsystem
  rate cmd select : Subsystem
  vel cmd select : Subsystem
  control_input : Outport  OutDataType=sfix(16)  OutScaling=2^0
  wires:
  Multiport Switch/1 -> Bus Creator1/4  "command"
  pos cmd select/1(pos_cmd) -> Multiport Switch/6
  att cmd select/1(att_cmd) -> Multiport Switch/4
  rate cmd select/1(rate_cmd) -> Multiport Switch/3
  Bus Selector/1 -> Multiport Switch/2
  Bus Selector4/3 -> Multiport Switch/1, Bus Creator1/3  "<CLAW_mode>"
  cmd_bus/1 -> pos cmd select/1(cmd_bus), vel cmd select/1(cmd_bus), Bus Selector4/1, Bus Selector/1, rate cmd select/1(cmd_bus), att cmd select/1(cmd_bus)
  vel cmd select/1(vel_cmd) -> Multiport Switch/5
  Bus Selector4/2 -> Bus Creator1/2  "<accel_submode>"
  Bus Selector4/1 -> Bus Creator1/1  "<full_surf_cmd>"
  Bus Creator1/1 -> control_input/1

== system main_sim_adapt_Gref_SP/control input (modified)/control input/generate commands/pos cmd generator ==
  cmd_bus : Inport  OutDataType=sfix(16)  OutScaling=2^0
  From Workspace5 : FromWorkspace  VariableName=pos_cmd_fw  SampleTime=MACH.dt  OutputAfterFinalValue=Holding final value
  Ground : Ground
  Multiport Switch2 : MultiPortSwitch  Inputs=4  zeroidx=on  SaturateOnIntegerOverflow=on
  circle pos cmd : Subsystem
  ramp pos cmd : Subsystem
  use_cam_rate_cmd1 : Constant  Value=pos_cmd_select  OutDataType=sfix(16)  OutScaling=2^0
  pos_cmd : Outport  OutDataType=sfix(16)  OutScaling=2^0
  wires:
  Ground/1 -> Multiport Switch2/2
  From Workspace5/1 -> Multiport Switch2/3
  use_cam_rate_cmd1/1 -> Multiport Switch2/1
  Multiport Switch2/1 -> pos_cmd/1
  ramp pos cmd/1(pos_cmd) -> Multiport Switch2/4
  circle pos cmd/1(pos_cmd) -> Multiport Switch2/5
  cmd_bus/1 -> ramp pos cmd/1(cmd_bus), circle pos cmd/1(cmd_bus)

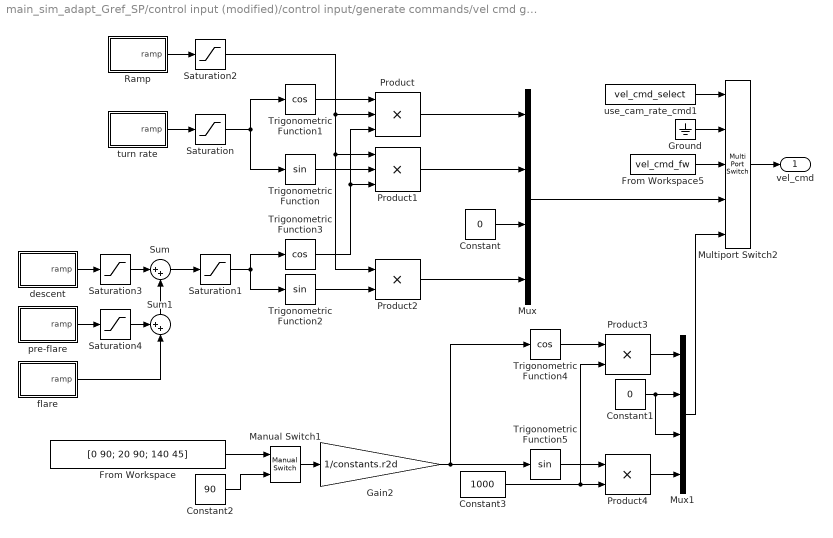
== system main_sim_adapt_Gref_SP/control input (modified)/control input/generate commands/vel cmd generator ==
  Constant : Constant  Value=0  OutDataType=sfix(16)  OutScaling=2^0
  Constant1 : Constant  Value=0  OutDataType=sfix(16)  OutScaling=2^0
  Constant2 : Constant  Value=90  OutDataType=sfix(16)  OutScaling=2^0
  Constant3 : Constant  Value=1000  OutDataType=sfix(16)  OutScaling=2^0
  From Workspace : FromWorkspace  VariableName=[0 90; 20 90; 140 45]  SampleTime=MACH.dt  OutputAfterFinalValue=Holding final value
  From Workspace5 : FromWorkspace  VariableName=vel_cmd_fw  SampleTime=MACH.dt  OutputAfterFinalValue=Holding final value
  Gain2 : Gain  Gain=1/constants.r2d  ParameterDataType=sfix(16)  ParameterScaling=2^0  OutDataType=sfix(16)  OutScaling=2^0
  Ground : Ground
  Manual Switch1 : simulink/Signal Routing/Manual Switch  SystemSampleTime=-1  sw=1  action=0  varsize=off
  Multiport Switch2 : MultiPortSwitch  Inputs=4  zeroidx=on  SaturateOnIntegerOverflow=on
  Mux : Mux
  Mux1 : Mux
  Product : Product  Inputs=3  OutDataType=sfix(16)  OutScaling=2^0  SaturateOnIntegerOverflow=on  OutDataTypeStr=Inherit: Same as first input
  Product1 : Product  Inputs=3  OutDataType=sfix(16)  OutScaling=2^0  SaturateOnIntegerOverflow=on  OutDataTypeStr=Inherit: Same as first input
  Product2 : Product  OutDataType=sfix(16)  OutScaling=2^0  SaturateOnIntegerOverflow=on  OutDataTypeStr=Inherit: Same as first input
  Product3 : Product  OutDataType=sfix(16)  OutScaling=2^0  SaturateOnIntegerOverflow=on  OutDataTypeStr=Inherit: Same as first input
  Product4 : Product  OutDataType=sfix(16)  OutScaling=2^0  SaturateOnIntegerOverflow=on  OutDataTypeStr=Inherit: Same as first input
  Ramp : Subsystem  mask{slope=accel_cmd, start_time=time_accel_cmd, initial_output=Nd_trim_IC, sample_time=MACH.dt}
      mask prompts: start_time "Start time:"; initial_output "Initial output:"; sample_time "Sample time (-1 for inherited):"
  Saturation : Saturate  UpperLimit=max_chi_cmd  LowerLimit=min_chi_cmd
  Saturation1 : Saturate  UpperLimit=0  LowerLimit=gam_cmd_descent
  Saturation2 : Saturate  UpperLimit=max_vel_cmd  LowerLimit=min_vel_cmd
  Saturation3 : Saturate  UpperLimit=0  LowerLimit=gam_cmd_descent
  Saturation4 : Saturate  UpperLimit=-gam_cmd_descent + gam_cmd_preflare  LowerLimit=-inf
  Sum : Sum  Inputs=|++  OutDataType=sfix(16)  OutScaling=2^0
  Sum1 : Sum  Orientation=up  Inputs=++|  OutDataType=sfix(16)  OutScaling=2^0
  Trigonometric Function : Trigonometry
  Trigonometric Function1 : Trigonometry  Operator=cos
  Trigonometric Function2 : Trigonometry
  Trigonometric Function3 : Trigonometry  Operator=cos
  Trigonometric Function4 : Trigonometry  Operator=cos
  Trigonometric Function5 : Trigonometry
  descent : Subsystem  mask{slope=gamdot_cmd_descent, start_time=time_gamdot_cmd_descent, initial_output=0, sample_time=MACH.dt}
      mask prompts: start_time "Start time:"; initial_output "Initial output:"; sample_time "Sample time (-1 for inherited):"
  flare : Subsystem  mask{slope=gamdot_cmd_flare, start_time=time_gamdot_cmd_flare, initial_output=0, sample_time=MACH.dt}
      mask prompts: start_time "Start time:"; initial_output "Initial output:"; sample_time "Sample time (-1 for inherited):"
  pre-flare : Subsystem  mask{slope=gamdot_cmd_preflare, start_time=time_gamdot_cmd_preflare, initial_output=0, sample_time=MACH.dt}
      mask prompts: start_time "Start time:"; initial_output "Initial output:"; sample_time "Sample time (-1 for inherited):"
  turn rate : Subsystem  mask{slope=turn_rate_cmd, start_time=time_turn_cmd, initial_output=0, sample_time=MACH.dt}
      mask prompts: start_time "Start time:"; initial_output "Initial output:"; sample_time "Sample time (-1 for inherited):"
  use_cam_rate_cmd1 : Constant  Value=vel_cmd_select  OutDataType=sfix(16)  OutScaling=2^0
  vel_cmd : Outport  OutDataType=sfix(16)  OutScaling=2^0
  wires:
  Trigonometric Function1/1 -> Product/1
  Trigonometric Function/1 -> Product1/2
  turn rate/1(ramp) -> Saturation/1
  Saturation/1 -> Trigonometric Function1/1, Trigonometric Function/1
  Product/1 -> Mux/1
  Product1/1 -> Mux/2
  Ramp/1(ramp) -> Saturation2/1
  Saturation1/1 -> Trigonometric Function3/1, Trigonometric Function2/1
  Trigonometric Function3/1 -> Product/3, Product1/3
  Product2/1 -> Mux/4
  Trigonometric Function2/1 -> Product2/2
  Saturation2/1 -> Product/2, Product1/1, Product2/1
  descent/1(ramp) -> Saturation3/1
  Sum/1 -> Saturation1/1
  Saturation3/1 -> Sum/1
  Constant/1 -> Mux/3
  pre-flare/1(ramp) -> Saturation4/1
  Sum1/1 -> Sum/2
  flare/1(ramp) -> Sum1/2
  Saturation4/1 -> Sum1/1
  Multiport Switch2/1 -> vel_cmd/1
  Constant1/1 -> Mux1/2, Mux1/3
  Trigonometric Function4/1 -> Product3/1
  Product3/1 -> Mux1/1
  Trigonometric Function5/1 -> Product4/1
  Product4/1 -> Mux1/4
  Mux1/1 -> Multiport Switch2/5
  Gain2/1 -> Trigonometric Function4/1, Trigonometric Function5/1
  Manual Switch1/1 -> Gain2/1
  From Workspace/1 -> Manual Switch1/1
  Constant2/1 -> Manual Switch1/2
  Mux/1 -> Multiport Switch2/4
  use_cam_rate_cmd1/1 -> Multiport Switch2/1
  From Workspace5/1 -> Multiport Switch2/3
  Constant3/1 -> Product4/2, Product3/2
  Ground/1 -> Multiport Switch2/2

== system main_sim_adapt_Gref_SP/control input (modified)/ideal responses/ideal att rate response/att loop ==
  e_cmd : Inport  OutDataType=sfix(16)  OutScaling=2^0
  e : Inport  Port=2  OutDataType=sfix(16)  OutScaling=2^0
  Discrete-Time Integrator : DiscreteIntegrator  IntegratorMethod=Integration: Backward Euler  InitialCondition=MACH_att_int_IC  SampleTime=-1  OutDataType=sfix(16)  OutScaling=2^0  ICPrevOutput=DiscIntNeverNeededParam  ICPrevScaledInput=DiscIntNeverNeededParam
  Gain1 : Gain  Gain=MACH_att_Kb  ParameterDataType=sfix(16)  ParameterScaling=2^0  OutDataType=sfix(16)  OutScaling=2^0  SaturateOnIntegerOverflow=on  OutDataTypeStr=Inherit: Same as input  ParamDataTypeStr=Inherit: Same as input
  Gain4 : Gain  Gain=MACH_att_Kc  ParameterDataType=sfix(16)  ParameterScaling=2^0  OutDataType=sfix(16)  OutScaling=2^0  SaturateOnIntegerOverflow=on  OutDataTypeStr=Inherit: Same as input  ParamDataTypeStr=Inherit: Same as input
  Gain5 : Gain  Gain=MACH_att_Ki.*MACH_att_Kb  ParameterDataType=sfix(16)  ParameterScaling=2^0  OutDataType=sfix(16)  OutScaling=2^0  SaturateOnIntegerOverflow=on  OutDataTypeStr=Inherit: Same as input  ParamDataTypeStr=Inherit: Same as input
  Sum2 : Sum  Inputs=|+-  OutDataType=sfix(16)  OutScaling=2^0  SaturateOnIntegerOverflow=on  InputSameDT=on  OutDataTypeStr=Inherit: Same as first input
  Sum3 : Sum  Inputs=++-  OutDataType=sfix(16)  OutScaling=2^0  SaturateOnIntegerOverflow=on  InputSameDT=on  OutDataTypeStr=Inherit: Same as first input
  Terminator : Terminator
  getedinv : utility_lib/getedinv  SystemSampleTime=-1
  pqr_cmd : Outport  OutDataType=sfix(16)  OutScaling=2^0
  wires:
  Gain1/1 -> getedinv/1
  Gain5/1 -> Discrete-Time Integrator/1
  Discrete-Time Integrator/1 -> Sum3/2
  Gain4/1 -> Sum3/1
  Sum3/1 -> Gain1/1
  Sum2/1 -> Gain5/1
  e_cmd/1 -> Sum2/1, Gain4/1
  getedinv/1 -> pqr_cmd/1
  e/1 -> Sum2/2, Sum3/3, getedinv/2
  getedinv/2 -> Terminator/1

== system main_sim_adapt_Gref_SP/control input (modified)/ideal responses/ideal att rate response/get att cmd ==
  note: Note: So that we can switch between a pqr command
      | and a quat command, the 4th component of command (throt)
      | is left until after the switch, and removed later.
  control_input : Inport  OutDataType=sfix(16)  OutScaling=2^0
  e : Inport  Port=2  OutDataType=sfix(16)  OutScaling=2^0
  Bus Selector1 : BusSelector  OutputSignals=mode_sw.CLAW_mode,command
  Constant1 : Constant  Value=[0 0 0 0]  OutDataType=sfix(16)  OutScaling=2^0
  Constant2 : Constant  Value=[5 6 7 8]  OutDataType=sfix(16)  OutScaling=2^0
  Constant3 : Constant  Value=[4 5 6]  OutDataType=sfix(16)  OutScaling=2^0
  Constant4 : Constant  Value=[1 2 3]  OutDataType=sfix(16)  OutScaling=2^0
  Constant5 : Constant  Value=[1 2 3 4]  OutDataType=sfix(16)  OutScaling=2^0
  Multiport Switch1 : MultiPortSwitch  Inputs=6  zeroidx=on
  Multiport Switch2 : MultiPortSwitch  Inputs=6  zeroidx=on
  Multiport Switch3 : MultiPortSwitch  Inputs=6  zeroidx=on
  convert to quat : Subsystem
  quatpqr_cmd : Outport  OutDataType=sfix(16)  OutScaling=2^0
  quat_select : Outport  Port=2  OutDataType=sfix(16)  OutScaling=2^0
  pqr_select : Outport  Port=3  OutDataType=sfix(16)  OutScaling=2^0
  wires:
  control_input/1 -> Bus Selector1/1
  Multiport Switch1/1 -> quatpqr_cmd/1
  Bus Selector1/1 -> Multiport Switch1/1, Multiport Switch2/1, Multiport Switch3/1  "<CLAW_mode>"
  Constant1/1 -> Multiport Switch1/2, Multiport Switch1/5, Multiport Switch1/6, Multiport Switch1/7
  Multiport Switch2/1 -> quat_select/1
  Multiport Switch3/1 -> pqr_select/1
  Constant2/1 -> Multiport Switch2/2, Multiport Switch2/3, Multiport Switch2/5, Multiport Switch2/6, Multiport Switch2/7
  Constant3/1 -> Multiport Switch3/2, Multiport Switch3/4, Multiport Switch3/5, Multiport Switch3/6, Multiport Switch3/7
  Bus Selector1/2 -> Multiport Switch1/3, convert to quat/1(att_cmd)  "<command>"
  Constant5/1 -> Multiport Switch2/4
  convert to quat/1(e_cmd) -> Multiport Switch1/4
  Constant4/1 -> Multiport Switch3/3
  e/1 -> convert to quat/2(e)

== system main_sim_adapt_Gref_SP/control input (modified)/ideal responses/ideal att rate response/rate loop ==
  pqr_cmd : Inport  OutDataType=sfix(16)  OutScaling=2^0
  pqr : Inport  Port=2  OutDataType=sfix(16)  OutScaling=2^0
  Discrete-Time Integrator : DiscreteIntegrator  IntegratorMethod=Integration: Backward Euler  InitialCondition=MACH_pqr_int_IC  SampleTime=-1  OutDataType=sfix(16)  OutScaling=2^0  ICPrevOutput=DiscIntNeverNeededParam  ICPrevScaledInput=DiscIntNeverNeededParam
  Gain : Gain  Gain=MACH_pqr_Kb  ParameterDataType=sfix(16)  ParameterScaling=2^0  OutDataType=sfix(16)  OutScaling=2^0  SaturateOnIntegerOverflow=on  OutDataTypeStr=Inherit: Same as input  ParamDataTypeStr=Inherit: Same as input
  Gain2 : Gain  Gain=0*MACH_pqr_Kc  ParameterDataType=sfix(16)  ParameterScaling=2^0  OutDataType=sfix(16)  OutScaling=2^0  SaturateOnIntegerOverflow=on  OutDataTypeStr=Inherit: Same as input  ParamDataTypeStr=Inherit: Same as input
  Gain3 : Gain  Gain=MACH_pqr_Ki.*MACH_pqr_Kb  ParameterDataType=sfix(16)  ParameterScaling=2^0  OutDataType=sfix(16)  OutScaling=2^0  SaturateOnIntegerOverflow=on  OutDataTypeStr=Inherit: Same as input  ParamDataTypeStr=Inherit: Same as input
  Sum : Sum  Inputs=|+-  OutDataType=sfix(16)  OutScaling=2^0  SaturateOnIntegerOverflow=on  InputSameDT=on  OutDataTypeStr=Inherit: Same as first input
  Sum1 : Sum  Inputs=++-  OutDataType=sfix(16)  OutScaling=2^0  SaturateOnIntegerOverflow=on  InputSameDT=on  OutDataTypeStr=Inherit: Same as first input
  pqrdot : Outport  OutDataType=sfix(16)  OutScaling=2^0
  wires:
  Sum/1 -> Gain3/1
  pqr_cmd/1 -> Gain2/1, Sum/1
  Gain/1 -> pqrdot/1
  Sum1/1 -> Gain/1
  Gain2/1 -> Sum1/1
  Discrete-Time Integrator/1 -> Sum1/2
  Gain3/1 -> Discrete-Time Integrator/1
  pqr/1 -> Sum/2, Sum1/3
